simulink model "FOC"  (R2021a)
settings: Solver=VariableStepAuto  StartTime=0.0  StopTime=10.0  RelTol=1e-3
libraries: mcbcontrolslib x2, pid_lib x2, mcbplantlib x1, simulink x1, autolibpmsmexterior x1
settings Model: Creator=hjt88  LastModifiedBy=hjt88

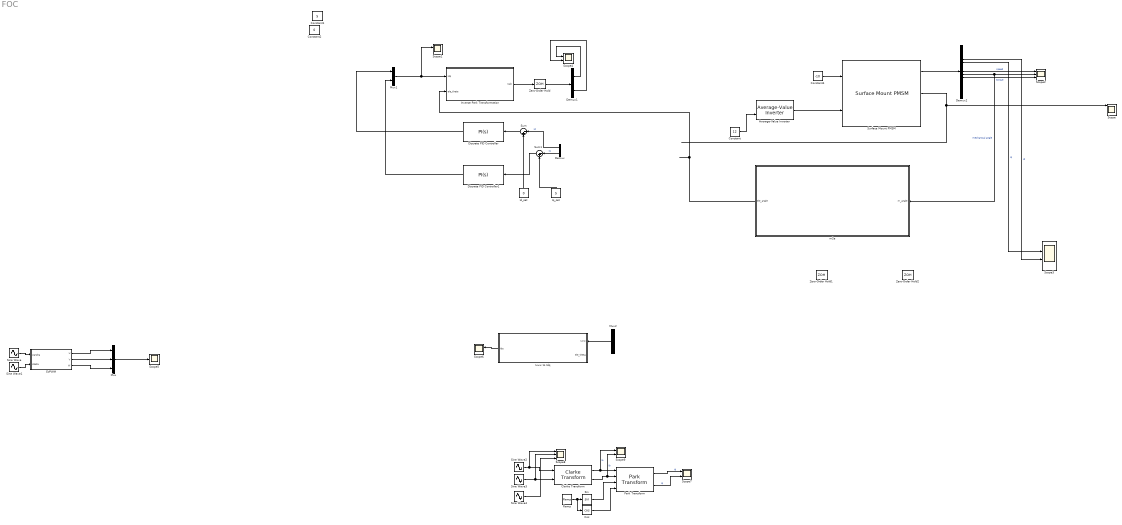
== system FOC ==
  Average-Value Inverter : mcbplantlib/Average-Value Inverter
  Clarke Transform : mcbcontrolslib/Clarke Transform  VariantControl=Variant2
  Constant : Constant  Value=12
  Constant1 : Constant  Value=5
  Constant2 : Constant  Value=0
  Constant4 : Constant  Value=-10
  Cos : Trigonometry  Operator=cos
  Demux : Demux  Outputs=2
  Demux1 : Demux  Outputs=2
  Demux2 : Demux  Outputs=15
  Discrete PID Controller : pid_lib/PID Controller  Controller=PI  Form=Parallel  TimeDomain=Continuous-time  UseExternalTs=off  SampleTime=-1  IntegratorMethod=Forward Euler  FilterMethod=Forward Euler  ControllerParametersSource=internal  P=0.395  I=0  D=0  UseFilter=on  N=100  TunerSelectOption=Transfer Function Based (PID Tuner App)  InitialConditionSource=internal  InitialConditionForIntegrator=0  InitialConditionForFilter=0  DifferentiatorICPrevScaledInput=0  ExternalReset=none  TrackingMode=off  Kt=1  LimitOutput=on  SatLimitsSource=internal  UpperSaturationLimit=2000  LowerSaturationLimit=-2000  LinearizeAsGain=off  AntiWindupMode=none  Kb=1  POutMin=[]  POutMax=[]  IOutMin=[]  IOutMax=[]  DOutMin=[]  DOutMax=[]  NOutMin=[]  NOutMax=[]  SumOutMin=[]  SumOutMax=[]  SaturationOutMin=[]  SaturationOutMax=[]  PParamMin=[]  PParamMax=[]  IParamMin=[]  IParamMax=[]  DParamMin=[]  DParamMax=[]  NParamMin=[]  NParamMax=[]  KbParamMin=[]  KbParamMax=[]  KtParamMin=[]  KtParamMax=[]  KbOutMin=[]  KbOutMax=[]  KtOutMin=[]  KtOutMax=[]  IntegratorOutMin=[]  IntegratorOutMax=[]  FilterOutMin=[]  FilterOutMax=[]  SumI1OutMin=[]  SumI1OutMax=[]  SumI2OutMin=[]  SumI2OutMax=[]  SumI3OutMin=[]  SumI3OutMax=[]  SumI4OutMin=[]  SumI4OutMax=[]  SumDOutMin=[]  SumDOutMax=[]  DifferentiatorOutMin=[]  DifferentiatorOutMax=[]  FilterDiffOutCoefMin=[]  FilterDiffOutCoefMax=[]  ReciprocalOutMin=[]  ReciprocalOutMax=[]  SumDenOutMin=[]  SumDenOutMax=[]  SumNumOutMin=[]  SumNumOutMax=[]  DivideOutMin=[]  DivideOutMax=[]  UdiffTsProdOutMin=[]  UdiffTsProdOutMax=[]  NTsProdOutMin=[]  NTsProdOutMax=[]  UintegralTsProdOutMin=[]  UintegralTsProdOutMax=[]  UngainTsProdOutMin=[]  UngainTsProdOutMax=[]  IntegratorContinuousStateAttributes=''  IntegratorStateMustResolveToSignalObject=off  IntegratorRTWStateStorageClass=Auto  FilterContinuousStateAttributes=''  FilterStateMustResolveToSignalObject=off  FilterRTWStateStorageClass=Auto  ParallelPVariant=InternalParameters  IdealPVariant=Disabled  IVariant=InternalParameters  DVariant=Disabled  IntegratorVariant=Continuous  SatVariant=Enabled  AWVariant=Passthrough  PCopyVariant=Disabled  TRVariant=Disabled  FdbkBlocksVariant=Forward  IdealPFdbkVariant=Disabled  SatFdbkVariant=Disabled  DerivativeFilterVariant=Disabled  NVariant=Disabled  NCopyVariant=Disabled_SignalSpec  FilterICVariant=Disabled  IntegratorICVariant=InternalICs  ExternalResetVariant=Disabled  TRSumVariant=Passthrough  SumFdbkVariant=Disabled  SumVariant=Sum_PI  TsampFilterVariant=InternalTs  TsampNgainVariant=Passthrough  TsampIntegralVariant=Passthrough  ExternalSaturationOutDataTypeStr=Inherit: Same as second input
  Discrete PID Controller1 : pid_lib/PID Controller  Controller=PI  Form=Parallel  TimeDomain=Continuous-time  UseExternalTs=off  SampleTime=-1  IntegratorMethod=Forward Euler  FilterMethod=Forward Euler  ControllerParametersSource=internal  P=0.395  I=0  D=0  UseFilter=on  N=100  TunerSelectOption=Transfer Function Based (PID Tuner App)  InitialConditionSource=internal  InitialConditionForIntegrator=0  InitialConditionForFilter=0  DifferentiatorICPrevScaledInput=0  ExternalReset=none  TrackingMode=off  Kt=1  LimitOutput=on  SatLimitsSource=internal  UpperSaturationLimit=20  LowerSaturationLimit=-20  LinearizeAsGain=on  AntiWindupMode=none  Kb=1  POutMin=[]  POutMax=[]  IOutMin=[]  IOutMax=[]  DOutMin=[]  DOutMax=[]  NOutMin=[]  NOutMax=[]  SumOutMin=[]  SumOutMax=[]  SaturationOutMin=[]  SaturationOutMax=[]  PParamMin=[]  PParamMax=[]  IParamMin=[]  IParamMax=[]  DParamMin=[]  DParamMax=[]  NParamMin=[]  NParamMax=[]  KbParamMin=[]  KbParamMax=[]  KtParamMin=[]  KtParamMax=[]  KbOutMin=[]  KbOutMax=[]  KtOutMin=[]  KtOutMax=[]  IntegratorOutMin=[]  IntegratorOutMax=[]  FilterOutMin=[]  FilterOutMax=[]  SumI1OutMin=[]  SumI1OutMax=[]  SumI2OutMin=[]  SumI2OutMax=[]  SumI3OutMin=[]  SumI3OutMax=[]  SumI4OutMin=[]  SumI4OutMax=[]  SumDOutMin=[]  SumDOutMax=[]  DifferentiatorOutMin=[]  DifferentiatorOutMax=[]  FilterDiffOutCoefMin=[]  FilterDiffOutCoefMax=[]  ReciprocalOutMin=[]  ReciprocalOutMax=[]  SumDenOutMin=[]  SumDenOutMax=[]  SumNumOutMin=[]  SumNumOutMax=[]  DivideOutMin=[]  DivideOutMax=[]  UdiffTsProdOutMin=[]  UdiffTsProdOutMax=[]  NTsProdOutMin=[]  NTsProdOutMax=[]  UintegralTsProdOutMin=[]  UintegralTsProdOutMax=[]  UngainTsProdOutMin=[]  UngainTsProdOutMax=[]  IntegratorContinuousStateAttributes=''  IntegratorStateMustResolveToSignalObject=off  IntegratorRTWStateStorageClass=Auto  FilterContinuousStateAttributes=''  FilterStateMustResolveToSignalObject=off  FilterRTWStateStorageClass=Auto  ParallelPVariant=InternalParameters  IdealPVariant=Disabled  IVariant=InternalParameters  DVariant=Disabled  IntegratorVariant=Continuous  SatVariant=Enabled  AWVariant=Passthrough  PCopyVariant=Disabled  TRVariant=Disabled  FdbkBlocksVariant=Forward  IdealPFdbkVariant=Disabled  SatFdbkVariant=Disabled  DerivativeFilterVariant=Disabled  NVariant=Disabled  NCopyVariant=Disabled_SignalSpec  FilterICVariant=Disabled  IntegratorICVariant=InternalICs  ExternalResetVariant=Disabled  TRSumVariant=Passthrough  SumFdbkVariant=Disabled  SumVariant=Sum_PI  TsampFilterVariant=InternalTs  TsampNgainVariant=Passthrough  TsampIntegralVariant=Passthrough  ExternalSaturationOutDataTypeStr=Inherit: Same as second input
  Id_set : Constant  Value=0
  Inverse Park Transformation : Subsystem
  Iq_set : Constant  Value=5
  Iuvw to Idq : Subsystem
  Mux : Mux  Inputs=3
  Mux1 : Mux  Inputs=2
  Mux2 : Mux  Inputs=3
  Park Transform : mcbcontrolslib/Park Transform  AxisAlignment=D-axis
      settings: SourceProductBaseCode=MT
  Ramp : simulink/Sources/Ramp  slope=-2*pi  start=0  InitialOutput=0
  SVPWM : Subsystem
  Scope : Scope  NumInputPorts=4
  Scope{1,4,6..7,9} (5 alike) : Scope  NumInputPorts=2
  Scope2 : Scope  NumInputPorts=3
  Scope3 : Scope  NumInputPorts=4
  Scope5 : Scope
  Scope8 : Scope  NumInputPorts=3
  Sin : Trigonometry
  Sine Wave : Sin  Amplitude=2  Frequency=3  SampleTime=0.01
  Sine Wave1 : Sin  Amplitude=2  Frequency=3  Phase=pi/2  SampleTime=0.01
  Sine Wave2 : Sin  Frequency=2*pi  SampleTime=0
  Sine Wave3 : Sin  Frequency=2*pi  Phase=2*pi/3  SampleTime=0
  Sine Wave4 : Sin  Frequency=2*pi  Phase=4*pi/3  SampleTime=0
  Sum : Sum  Inputs=|-+
  Sum1 : Sum  Inputs=|-+
  Surface Mount PMSM : autolibpmsmexterior/Surface Mount PMSM  port_config=Torque  sim_type=Continuous  Ts=0.001  P=11  Rs=7.8  Ldq_=3.95e-3  KConstText=Back-emf constant (Ke):  lambda_pm=0.2205  Ke=159.9771  Kt=0.2  mechanical=[0.0027, 4.924e-4, 0]  idq0=[0 0]  theta_init=0  omega_init=0  KConst=0.2205  lambda_pm_calc=0.080182  RefBlkName='autolibpmsmexterior/Surface Mount PMSM'  aMode=5  Ldq="[0.0017      0.0017]"
      settings: SourceProductBaseCode=PW,DR,MT,UV,VE
  Zero-Order Hold : ZeroOrderHold  SampleTime=0.0005
  Zero-Order Hold1 : ZeroOrderHold  SampleTime=0.0005
  Zero-Order Hold2 : ZeroOrderHold  SampleTime=0.0005
  m2e : Subsystem
  wires:
  Average-Value Inverter/1 -> Surface Mount PMSM/2
  Constant/1 -> Average-Value Inverter/2
  SVPWM/2(V) -> Mux/2
  SVPWM/1(U) -> Mux/1
  SVPWM/3(W) -> Mux/3
  Mux/1 -> Scope5/1
  ? -> Scope3/1, Demux/1
  Sum/1 -> Discrete PID Controller/1
  Demux/1 -> Sum/1  "Id"
  Id_set/1 -> Sum/2
  Sum1/1 -> Discrete PID Controller1/1
  Demux/2 -> Sum1/1  "Iq"
  Iq_set/1 -> Sum1/2
  Mux1/1 -> Scope1/1, Inverse Park Transformation/1(Idq)
  Surface Mount PMSM/1 -> Demux2/1
  Demux2/8 -> Scope2/1  "speed"
  Demux2/9 -> m2e/1(m_angle), Scope2/2  "mechanical angle"
  Demux2/10 -> Scope2/3  "torque"
  m2e/1(ele_angle) -> Inverse Park Transformation/2(ele_theta)
  Demux1/1 -> Scope4/1
  Demux1/2 -> Scope4/2
  Surface Mount PMSM/2 -> Scope/1
  Zero-Order Hold/1 -> Demux1/1
  Inverse Park Transformation/1(Uab) -> Zero-Order Hold/1
  Demux2/4 -> Scope3/3  "Id"
  Demux2/5 -> Scope3/2  "Iq"
  Discrete PID Controller/1 -> Mux1/1
  Discrete PID Controller1/1 -> Mux1/2
  Constant4/1 -> Surface Mount PMSM/1
  Mux2/1 -> Iuvw to Idq/1(Iuvw)
  Iuvw to Idq/1(Idq) -> Scope6/1
  Clarke Transform/1 -> Scope9/1, Park Transform/1  "Ia"
  Clarke Transform/2 -> Scope9/2, Park Transform/2  "Ib"
  Sine Wave2/1 -> Scope8/1, Clarke Transform/1
  Sine Wave3/1 -> Scope8/2, Clarke Transform/2
  Ramp/1 -> Cos/1, Sin/1
  Sin/1 -> Park Transform/3
  Cos/1 -> Park Transform/4
  Park Transform/1 -> Scope7/1  "Id"
  Park Transform/2 -> Scope7/2  "Iq"
  Sine Wave4/1 -> Scope8/3
  Sine Wave/1 -> SVPWM/1(Uarpha)
  Sine Wave1/1 -> SVPWM/2(Ubeta)

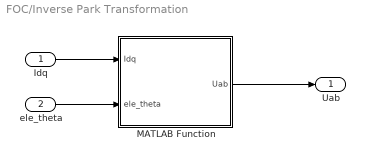
== system FOC/Inverse Park Transformation ==
  Idq : Inport
  ele_theta : Inport  Port=2
  MATLAB Function : MATLAB Function  TreatAsAtomicUnit=on
  Uab : Outport
  wires:
  MATLAB Function/1(Uab) -> Uab/1
  Idq/1 -> MATLAB Function/1(Idq)
  ele_theta/1 -> MATLAB Function/2(ele_theta)

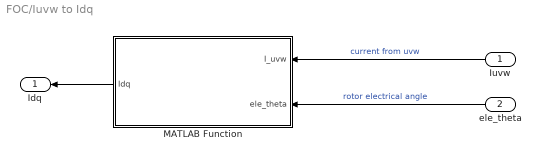
== system FOC/Iuvw to Idq ==
  Iuvw : Inport
  ele_theta : Inport  Port=2
  MATLAB Function : MATLAB Function  TreatAsAtomicUnit=on
  Idq : Outport
  wires:
  Iuvw/1 -> MATLAB Function/1(I_uvw)  "current from uvw"
  ele_theta/1 -> MATLAB Function/2(ele_theta)  "rotor electrical angle"
  MATLAB Function/1(Idq) -> Idq/1

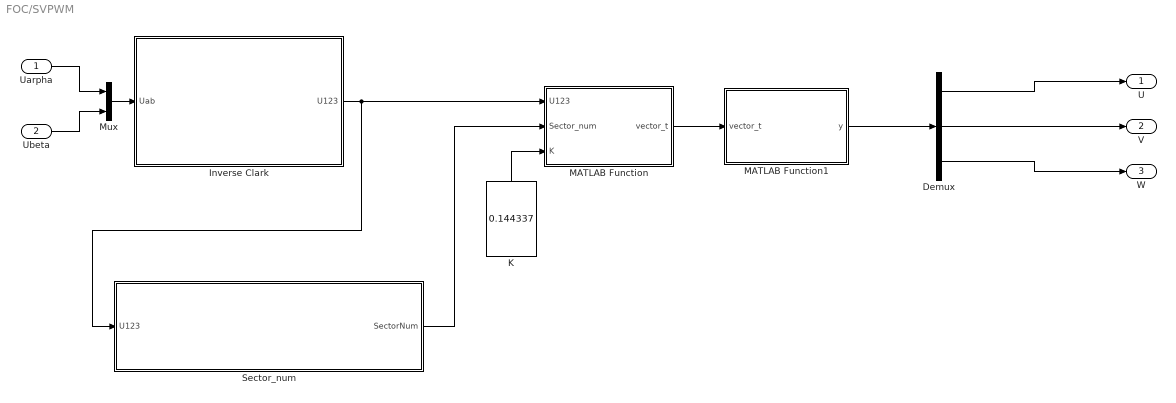
== system FOC/SVPWM ==
  Uarpha : Inport
  Ubeta : Inport  Port=2
  Demux : Demux  Outputs=3
  Inverse Clark : Subsystem
  K : Constant  Value=0.144337
  MATLAB Function : MATLAB Function  TreatAsAtomicUnit=on
  MATLAB Function1 : MATLAB Function  TreatAsAtomicUnit=on
  Mux : Mux  Inputs=2
  Sector_num : Subsystem
  U : Outport
  V : Outport  Port=2
  W : Outport  Port=3
  wires:
  Uarpha/1 -> Mux/1
  Ubeta/1 -> Mux/2
  Demux/2 -> V/1
  Demux/1 -> U/1
  Demux/3 -> W/1
  Mux/1 -> Inverse Clark/1(Uab)
  Inverse Clark/1(U123) -> MATLAB Function/1(U123), Sector_num/1(U123)
  Sector_num/1(SectorNum) -> MATLAB Function/2(Sector_num)
  K/1 -> MATLAB Function/3(K)
  MATLAB Function/1(vector_t) -> MATLAB Function1/1(vector_t)
  MATLAB Function1/1(y) -> Demux/1

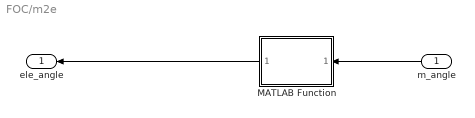
== system FOC/m2e ==
  m_angle : Inport
  MATLAB Function : MATLAB Function  TreatAsAtomicUnit=on
  ele_angle : Outport
  wires:
  m_angle/1 -> MATLAB Function/1(m_angle)
  MATLAB Function/1(ele_angle) -> ele_angle/1

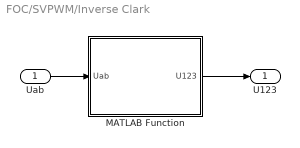
== system FOC/SVPWM/Inverse Clark ==
  Uab : Inport
  MATLAB Function : MATLAB Function  TreatAsAtomicUnit=on
  U123 : Outport
  wires:
  Uab/1 -> MATLAB Function/1(Uab)
  MATLAB Function/1(U123) -> U123/1

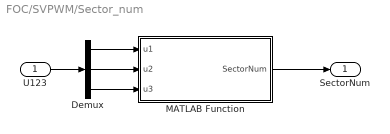
== system FOC/SVPWM/Sector_num ==
  U123 : Inport
  Demux : Demux  Outputs=3
  MATLAB Function : MATLAB Function  TreatAsAtomicUnit=on
  SectorNum : Outport
  wires:
  MATLAB Function/1(SectorNum) -> SectorNum/1
  U123/1 -> Demux/1
  Demux/1 -> MATLAB Function/1(u1)
  Demux/2 -> MATLAB Function/2(u2)
  Demux/3 -> MATLAB Function/3(u3)

== matlab function FOC/Iuvw to Idq/MATLAB Function ==
  data: I_uvw input; Idq output; ele_theta input
function Idq = fcn(I_uvw,ele_theta)
    cos_theta = cos(ele_theta);
    sin_theta = sin(ele_theta);
Idq =2/3* [cos_theta, -0.5*cos_theta+0.866*sin_theta, -0.866*sin_theta-0.5*cos_theta;
     -sin_theta, 0.5*sin_theta+0.866*cos_theta,  -0.866*cos_theta+0.5*sin_theta]*I_uvw;

== matlab function FOC/SVPWM/MATLAB Function ==
  data: U123 input; vector_t output; Sector_num input; K input
function vector_t= fcn(U123,Sector_num,K)
s_num = uint8(Sector_num);
vector_t = zeros(7,1);
vctable=[2,1;3,2;1,3;2,1;3,2;1,3];
temp1 = abs((K*U123(vctable(s_num,1),1)));
temp2 = abs(K*U123(vctable(s_num,2),1));
vector_t(s_num,1) = temp1;
vector_t((mod(s_num,6)+1),1) = temp2;
vector_t(7,1) = 0.5*(1-temp1-temp2);

== matlab function FOC/SVPWM/Inverse Clark/MATLAB Function ==
  data: Uab input; U123 output
function U123 = fcn(Uab)

U123 = [0,1;0.866,-0.5;-0.866,-0.5]*Uab;

== matlab function FOC/SVPWM/Sector_num/MATLAB Function ==
  data: u1 input; SectorNum output; u2 input; u3 input
function SectorNum = fcn(u1,u2,u3)
if u1>0
    A=1;
else 
    A=0;
end
if u2>0
    B=1;
else 
    B=0;
end
if u3>0
    C=1;
else 
    C=0;
end
N = 4 * C + 2 * B + A;
N2Sector = [2,6,1,4,3,5];
SectorNum = N2Sector(1,N);

== matlab function FOC/SVPWM/MATLAB Function1 ==
  data: vector_t input; y output
function y = fcn(vector_t)
V2T_Table=[1,1,0,0,0,1,1;
           0,1,1,1,0,0,1;
           0,0,0,1,1,1,1];
y = V2T_Table*vector_t;

== matlab function FOC/m2e/MATLAB Function ==
  data: m_angle input; ele_angle output
function ele_angle = fcn(m_angle)

ele_angle = mod(m_angle*11,2*pi);

== matlab function FOC/Inverse Park Transformation/MATLAB Function ==
  data: Idq input; Uab output; ele_theta input
function Uab = fcn(Idq,ele_theta)
    cos_theta = cos(ele_theta);
    sin_theta = sin(ele_theta);
Uab = [-sin_theta,cos_theta;
       cos_theta,sin_theta]*Idq;
